simulink model "Calculate_C2filterout"  (R2019b)
settings: Solver=FixedStepAuto  StartTime=0.0  StopTime=testtime  RelTol=1e-3
InitFcn:
  | AN_InitFcn_Callback
StopFcn:
  | AN_StopFcn_Callback
undefined symbols (not defined in the file or in its folder): cf
settings Model: Creator=mblun  LastModifiedBy=cb50701
settings DataIOCC: SaveOutput=off  SaveTime=off
settings OptimizationCC: BlockReduction=off  ConditionallyExecuteInputs=off  DefaultParameterBehavior=Inlined
settings SFSimCC: CustomCodeUndefinedFunction=UseInterfaceOnly

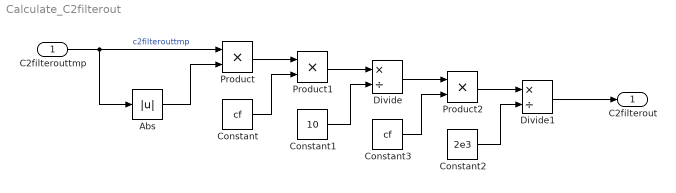
== system Calculate_C2filterout ==
  C2filterouttmp : Inport  OutDataTypeStr=double  PortDimensions=[1 1]  SampleTime=[2.0833333333333333e-05,0]
  Abs : Abs
  Constant : Constant  Value=cf  SampleTime=-1
  Constant1 : Constant  Value=10  SampleTime=-1
  Constant2 : Constant  Value=2e3  SampleTime=-1
  Constant3 : Constant  Value=cf  SampleTime=-1
  Divide : Product  Inputs=*/  SaturateOnIntegerOverflow=on  RndMeth=Zero
  Divide1 : Product  Inputs=*/  SaturateOnIntegerOverflow=on  RndMeth=Zero
  Product : Product
  Product1 : Product
  Product2 : Product
  C2filterout : Outport  OutDataTypeStr=double  PortDimensions=[1 1]  SampleTime=[2.0833333333333333e-05,0]  VectorParamsAs1DForOutWhenUnconnected=off
  wires:
  C2filterouttmp/1 -> Abs/1, Product/1  "c2filterouttmp"
  Abs/1 -> Product/2
  Product/1 -> Product1/1
  Constant/1 -> Product1/2
  Product1/1 -> Divide/1
  Constant1/1 -> Divide/2
  Product2/1 -> Divide1/1
  Constant2/1 -> Divide1/2
  Constant3/1 -> Product2/2
  Divide/1 -> Product2/1
  Divide1/1 -> C2filterout/1
